simulink model "GFM"  (R2021b)
settings: Solver=ode8  StartTime=0.0  StopTime=5  FixedStep=0.0001  RelTol=1e-3
libraries: spsFirstOrderFilterLib x7, slpidlib x4, spsThreePhaseSeriesRLCBranchLib x4, spsThreePhaseVIMeasurementLib x3, spsabctodq0Lib x3, spsGroundLib x2, rtlab x1, spsCurrentMeasurementLib x1, spsDCVoltageSourceLib x1, spsPower3phInstantaneousLib x1, spsSeriesRLCBranchLib x1, simulink x1
settings Model: Creator=Silov  LastModifiedBy=ti
settings SolverCC: AlgebraicLoopSolver=TrustRegion
settings OptimizationCC: BlockReduction=off  OptimizeBlockIOStorage=off
settings DebuggingCC: SFMachineParentedDataDiag=warning  ArithmeticOperatorsInVariantConditions=warning
settings SFSimCC: CustomCodeUndefinedFunction=UseInterfaceOnly

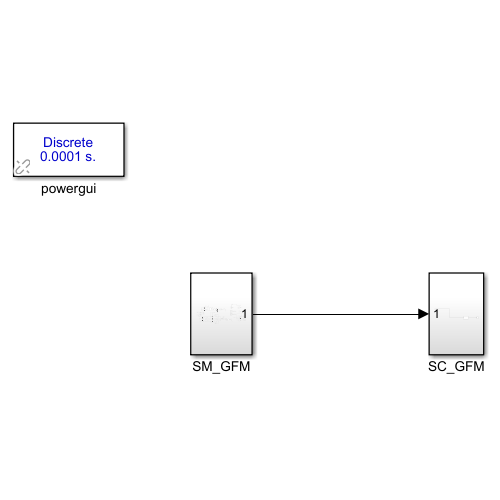
[thumbnail: Simulink's stored preview of the top-level diagram]
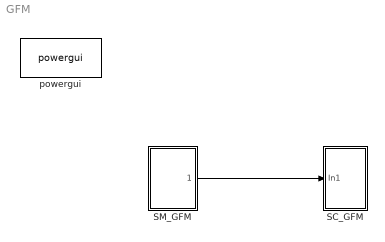
== system GFM ==
  SC_GFM : Subsystem
  SM_GFM : Subsystem
  powergui : spspowerguiLib/powergui  Priority=1  SimulationMode=Discrete  SampleTime=0.0001  frequency=60  Iterations=50  frequencyindice=0  Pbase=100e6  ErrMax=1e-4  UnitsV=kV  UnitsW=MW  buscounter=0  FunctionMessages=off  echomessages=off  EnableUseOfTLC=off  CurrentSourceSwitches=off  DisableSnubberDevices=off  DisableRonSwitches=off  DisableVfSwitches=off  DisplayEquations=off  AutomaticDiscreteSolvers=off  SolverType=Tustin/Backward Euler (TBE)  Interpol=off  ExternalGateDelay=off  methode=off  Ts=100  x0status=blocks  SPID=off  SwTol=0  HookPort=off  NonlinearTolerance=1e-4  nMaxIteration=100  ContinueOnMaxIteration=off  RestoreLinks=warning  ResistiveCurrentMeasurement=off  Frange=[0:2:500]  Ylog=off  Xlog=on  ShowGrid=off  save=off  variable=ZData  structure=grid_current  ZoomFFT=off  StartTime=0.5  cycles=1  DisplayStyle=2  fundamental=50  FreqAxis=off  MaxFrequency=1000  frequencyindicesteady=1  RmsSteady=1  display=off
  wires:
  SM_GFM/1(Outport) -> SC_GFM/1(In1)

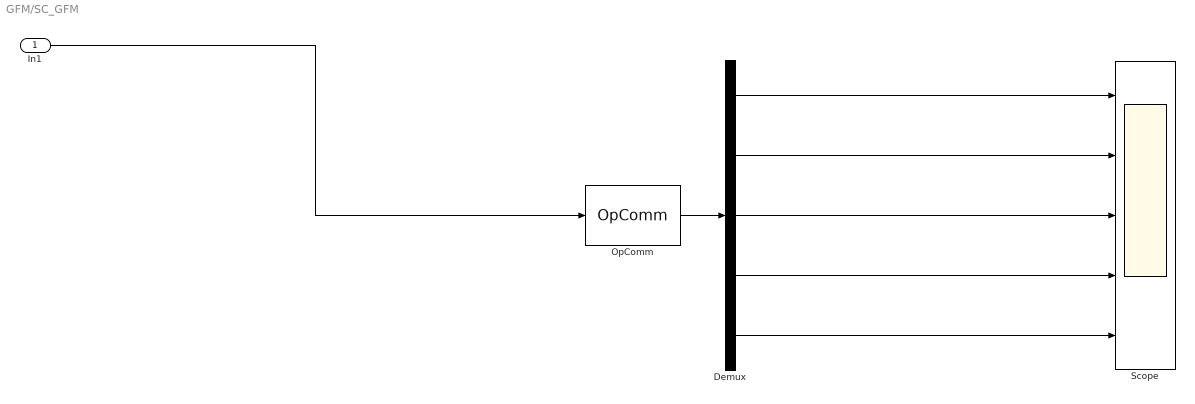
== system GFM/SC_GFM ==
  In1 : Inport
  Demux : Demux  Outputs=5
  OpComm : rtlab/OpComm  nbport=1  groupe_acq=1  subsys_rate=0  st=0  Synchronization=on  Interpolation=on  Threshold=1.0  Missed_Data=off  Sim_Time=off  Samples=off  dynSigOut=off  from_console=0  warning_done=off  writeOpCommFile=off  Offset=off
      settings: SourceProductName=RT-LAB
  Scope : Scope  NumInputPorts=5
  wires:
  OpComm/1 -> Demux/1
  In1/1 -> OpComm/1
  Demux/1 -> Scope/1
  Demux/2 -> Scope/2
  Demux/3 -> Scope/3
  Demux/4 -> Scope/4
  Demux/5 -> Scope/5

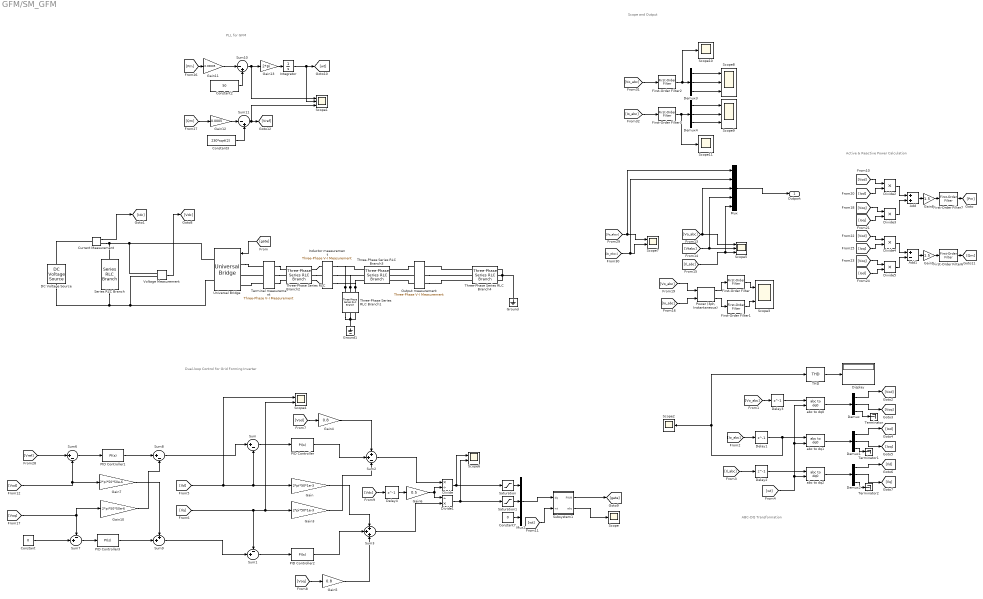
== system GFM/SM_GFM ==
  note: Dual-loop Control for Grid Forming Inverter
  note: ABC-DQ Transformation
  note: Active & Reactive Power Calculation
  note: Scope and Output
  note: PLL for GFM
  Add : Sum
  Add1 : Sum  Inputs=+-
  Constant : Constant  Value=0
  Constant2 : Constant  Value=50
  Constant3 : Constant  Value=230*sqrt(2)
  Constant7 : Constant  Value=0
  Current Measurement : spsCurrentMeasurementLib/Current Measurement  PhasorSimulation=off  OutputType=Complex  PSBequivalent=0
  DC Voltage Source : spsDCVoltageSourceLib/DC Voltage Source  Amplitude=750  Measurements=None
  Delay{1..4} (4 alike) : Delay  DelayLength=1
  Demux{,1..4} (5 alike) : Demux  Outputs=3
  Display : Display
  Divide : Product  Inputs=*/
  Divide1 : Product  Inputs=/*
  Divide{2..5} (4 alike) : Product  Inputs=**
  First-Order Filter{,1..3,6..7} (6 alike) : spsFirstOrderFilterLib/First-Order Filter  FilterType=Lowpass  Tc=0.03183  Ts=0  Initialize=off  Vac_Init=[0, 0, 60]  Vdc_Init=0  PlotResponse=off  FreqRange="[0,  200,  1]"
  Gain : Gain  Gain=2*pi*50*1e-3
  Gain10 : Gain  Gain=2*pi*50*50e-6
  Gain11 : Gain  Gain=0.00005
  Gain12 : Gain  Gain=0.0005
  Gain13 : Gain  Gain=2*pi
  Gain3 : Gain  Gain=2*pi*50*1e-3
  Gain4 : Gain  Gain=0.8
  Gain5 : Gain  Gain=0.8
  Gain6 : Gain  Gain=0.5
  Gain7 : Gain  Gain=2*pi*50*50e-6
  Gain8 : Gain  Gain=1.5
  Gain9 : Gain  Gain=1.5
  Ground : spsGroundLib/Ground  LConnTagsString=a
  Ground1 : spsGroundLib/Ground  LConnTagsString=a
  Inductor measurement : spsThreePhaseVIMeasurementLib/Three-Phase V-I Measurement  VoltageMeasurement=phase-to-ground  SetLabelV=on  LabelV=Vl_abc  Vpu=off  VpuLL=off  CurrentMeasurement=yes  SetLabelI=on  LabelI=Il_abc  Ipu=off  Pbase=100e6  Vbase=500e3  OutputType=Complex  PhasorSimulation=off  PSBequivalent=0
  Integrator : Integrator  WrapState=on  WrappedStateUpperValue=2*pi  WrappedStateLowerValue=0
  Mux : Mux  Inputs=5
  Mux2 : Mux  Inputs=3
  Output measurement : spsThreePhaseVIMeasurementLib/Three-Phase V-I Measurement  VoltageMeasurement=phase-to-ground  SetLabelV=on  LabelV=Vo_abc  Vpu=off  VpuLL=off  CurrentMeasurement=yes  SetLabelI=on  LabelI=Io_abc  Ipu=off  Pbase=100e6  Vbase=500e3  OutputType=Complex  PhasorSimulation=off  PSBequivalent=0
  PID Controller : slpidlib/PID Controller  Controller=PI  Form=Parallel  TimeDomain=Continuous-time  UseExternalTs=off  SampleTime=-1  IntegratorMethod=Forward Euler  FilterMethod=Forward Euler  ControllerParametersSource=internal  P=2*pi  I=pi*1000  D=0  UseFilter=on  N=100  TunerSelectOption=Transfer Function Based (PID Tuner App)  InitialConditionSource=internal  InitialConditionForIntegrator=0  InitialConditionForFilter=0  DifferentiatorICPrevScaledInput=0  ExternalReset=none  TrackingMode=off  Kt=1  LimitOutput=off  SatLimitsSource=internal  UpperSaturationLimit=inf  LowerSaturationLimit=-inf  LinearizeAsGain=on  AntiWindupMode=none  Kb=1  POutMin=[]  POutMax=[]  IOutMin=[]  IOutMax=[]  DOutMin=[]  DOutMax=[]  NOutMin=[]  NOutMax=[]  SumOutMin=[]  SumOutMax=[]  SaturationOutMin=[]  SaturationOutMax=[]  PParamMin=[]  PParamMax=[]  IParamMin=[]  IParamMax=[]  DParamMin=[]  DParamMax=[]  NParamMin=[]  NParamMax=[]  KbParamMin=[]  KbParamMax=[]  KtParamMin=[]  KtParamMax=[]  KbOutMin=[]  KbOutMax=[]  KtOutMin=[]  KtOutMax=[]  IntegratorOutMin=[]  IntegratorOutMax=[]  FilterOutMin=[]  FilterOutMax=[]  SumI1OutMin=[]  SumI1OutMax=[]  SumI2OutMin=[]  SumI2OutMax=[]  SumI3OutMin=[]  SumI3OutMax=[]  SumI4OutMin=[]  SumI4OutMax=[]  SumDOutMin=[]  SumDOutMax=[]  DifferentiatorOutMin=[]  DifferentiatorOutMax=[]  FilterDiffOutCoefMin=[]  FilterDiffOutCoefMax=[]  ReciprocalOutMin=[]  ReciprocalOutMax=[]  SumDenOutMin=[]  SumDenOutMax=[]  SumNumOutMin=[]  SumNumOutMax=[]  DivideOutMin=[]  DivideOutMax=[]  UdiffTsProdOutMin=[]  UdiffTsProdOutMax=[]  NTsProdOutMin=[]  NTsProdOutMax=[]  UintegralTsProdOutMin=[]  UintegralTsProdOutMax=[]  UngainTsProdOutMin=[]  UngainTsProdOutMax=[]  FilterDenConstantOutDataTypeStr=Inherit: Inherit via back propagation  FilterDenConstantOutMin=[]  FilterDenConstantOutMax=[]  PCopyOutDataTypeStr=Inherit: Inherit via back propagation  PCopyOutMin=[]  PCopyOutMax=[]  NCopyOutDataTypeStr=Inherit: Inherit via back propagation  NCopyOutMin=[]  NCopyOutMax=[]  IntegratorContinuousStateAttributes=''  IntegratorStateMustResolveToSignalObject=off  IntegratorRTWStateStorageClass=Auto  FilterContinuousStateAttributes=''  FilterStateMustResolveToSignalObject=off  FilterRTWStateStorageClass=Auto  ParallelPVariant=InternalParameters  IdealPVariant=Disabled  IVariant=InternalParameters  DVariant=Disabled  IntegratorVariant=Continuous  SatVariant=Disabled  AWVariant=Passthrough  PCopyVariant=Disabled  TRVariant=Disabled  FdbkBlocksVariant=Forward  IdealPFdbkVariant=Disabled  SatFdbkVariant=Disabled  DerivativeFilterVariant=Disabled  NVariant=Disabled  NCopyVariant=Disabled_SignalSpec  FilterICVariant=Disabled  IntegratorICVariant=InternalICs  ExternalResetVariant=Disabled  TRSumVariant=Passthrough  SumFdbkVariant=Disabled  SumVariant=Sum_PI  TsampFilterVariant=InternalTs  TsampNgainVariant=Passthrough  TsampIntegralVariant=Passthrough  ExternalSaturationOutDataTypeStr=Inherit: Same as second input
  PID Controller1 : slpidlib/PID Controller  Controller=PI  Form=Parallel  TimeDomain=Continuous-time  UseExternalTs=off  SampleTime=-1  IntegratorMethod=Forward Euler  FilterMethod=Forward Euler  ControllerParametersSource=internal  P=pi/100  I=20*pi  D=0  UseFilter=on  N=100  TunerSelectOption=Transfer Function Based (PID Tuner App)  InitialConditionSource=internal  InitialConditionForIntegrator=0  InitialConditionForFilter=0  DifferentiatorICPrevScaledInput=0  ExternalReset=none  TrackingMode=off  Kt=1  LimitOutput=off  SatLimitsSource=internal  UpperSaturationLimit=inf  LowerSaturationLimit=-inf  LinearizeAsGain=on  AntiWindupMode=none  Kb=1  POutMin=[]  POutMax=[]  IOutMin=[]  IOutMax=[]  DOutMin=[]  DOutMax=[]  NOutMin=[]  NOutMax=[]  SumOutMin=[]  SumOutMax=[]  SaturationOutMin=[]  SaturationOutMax=[]  PParamMin=[]  PParamMax=[]  IParamMin=[]  IParamMax=[]  DParamMin=[]  DParamMax=[]  NParamMin=[]  NParamMax=[]  KbParamMin=[]  KbParamMax=[]  KtParamMin=[]  KtParamMax=[]  KbOutMin=[]  KbOutMax=[]  KtOutMin=[]  KtOutMax=[]  IntegratorOutMin=[]  IntegratorOutMax=[]  FilterOutMin=[]  FilterOutMax=[]  SumI1OutMin=[]  SumI1OutMax=[]  SumI2OutMin=[]  SumI2OutMax=[]  SumI3OutMin=[]  SumI3OutMax=[]  SumI4OutMin=[]  SumI4OutMax=[]  SumDOutMin=[]  SumDOutMax=[]  DifferentiatorOutMin=[]  DifferentiatorOutMax=[]  FilterDiffOutCoefMin=[]  FilterDiffOutCoefMax=[]  ReciprocalOutMin=[]  ReciprocalOutMax=[]  SumDenOutMin=[]  SumDenOutMax=[]  SumNumOutMin=[]  SumNumOutMax=[]  DivideOutMin=[]  DivideOutMax=[]  UdiffTsProdOutMin=[]  UdiffTsProdOutMax=[]  NTsProdOutMin=[]  NTsProdOutMax=[]  UintegralTsProdOutMin=[]  UintegralTsProdOutMax=[]  UngainTsProdOutMin=[]  UngainTsProdOutMax=[]  FilterDenConstantOutDataTypeStr=Inherit: Inherit via back propagation  FilterDenConstantOutMin=[]  FilterDenConstantOutMax=[]  PCopyOutDataTypeStr=Inherit: Inherit via back propagation  PCopyOutMin=[]  PCopyOutMax=[]  NCopyOutDataTypeStr=Inherit: Inherit via back propagation  NCopyOutMin=[]  NCopyOutMax=[]  IntegratorContinuousStateAttributes=''  IntegratorStateMustResolveToSignalObject=off  IntegratorRTWStateStorageClass=Auto  FilterContinuousStateAttributes=''  FilterStateMustResolveToSignalObject=off  FilterRTWStateStorageClass=Auto  ParallelPVariant=InternalParameters  IdealPVariant=Disabled  IVariant=InternalParameters  DVariant=Disabled  IntegratorVariant=Continuous  SatVariant=Disabled  AWVariant=Passthrough  PCopyVariant=Disabled  TRVariant=Disabled  FdbkBlocksVariant=Forward  IdealPFdbkVariant=Disabled  SatFdbkVariant=Disabled  DerivativeFilterVariant=Disabled  NVariant=Disabled  NCopyVariant=Disabled_SignalSpec  FilterICVariant=Disabled  IntegratorICVariant=InternalICs  ExternalResetVariant=Disabled  TRSumVariant=Passthrough  SumFdbkVariant=Disabled  SumVariant=Sum_PI  TsampFilterVariant=InternalTs  TsampNgainVariant=Passthrough  TsampIntegralVariant=Passthrough  ExternalSaturationOutDataTypeStr=Inherit: Same as second input
  PID Controller2 : slpidlib/PID Controller  Controller=PI  Form=Parallel  TimeDomain=Continuous-time  UseExternalTs=off  SampleTime=-1  IntegratorMethod=Forward Euler  FilterMethod=Forward Euler  ControllerParametersSource=internal  P=2*pi  I=pi*1000  D=0  UseFilter=on  N=100  TunerSelectOption=Transfer Function Based (PID Tuner App)  InitialConditionSource=internal  InitialConditionForIntegrator=0  InitialConditionForFilter=0  DifferentiatorICPrevScaledInput=0  ExternalReset=none  TrackingMode=off  Kt=1  LimitOutput=off  SatLimitsSource=internal  UpperSaturationLimit=inf  LowerSaturationLimit=-inf  LinearizeAsGain=on  AntiWindupMode=none  Kb=1  POutMin=[]  POutMax=[]  IOutMin=[]  IOutMax=[]  DOutMin=[]  DOutMax=[]  NOutMin=[]  NOutMax=[]  SumOutMin=[]  SumOutMax=[]  SaturationOutMin=[]  SaturationOutMax=[]  PParamMin=[]  PParamMax=[]  IParamMin=[]  IParamMax=[]  DParamMin=[]  DParamMax=[]  NParamMin=[]  NParamMax=[]  KbParamMin=[]  KbParamMax=[]  KtParamMin=[]  KtParamMax=[]  KbOutMin=[]  KbOutMax=[]  KtOutMin=[]  KtOutMax=[]  IntegratorOutMin=[]  IntegratorOutMax=[]  FilterOutMin=[]  FilterOutMax=[]  SumI1OutMin=[]  SumI1OutMax=[]  SumI2OutMin=[]  SumI2OutMax=[]  SumI3OutMin=[]  SumI3OutMax=[]  SumI4OutMin=[]  SumI4OutMax=[]  SumDOutMin=[]  SumDOutMax=[]  DifferentiatorOutMin=[]  DifferentiatorOutMax=[]  FilterDiffOutCoefMin=[]  FilterDiffOutCoefMax=[]  ReciprocalOutMin=[]  ReciprocalOutMax=[]  SumDenOutMin=[]  SumDenOutMax=[]  SumNumOutMin=[]  SumNumOutMax=[]  DivideOutMin=[]  DivideOutMax=[]  UdiffTsProdOutMin=[]  UdiffTsProdOutMax=[]  NTsProdOutMin=[]  NTsProdOutMax=[]  UintegralTsProdOutMin=[]  UintegralTsProdOutMax=[]  UngainTsProdOutMin=[]  UngainTsProdOutMax=[]  FilterDenConstantOutDataTypeStr=Inherit: Inherit via back propagation  FilterDenConstantOutMin=[]  FilterDenConstantOutMax=[]  PCopyOutDataTypeStr=Inherit: Inherit via back propagation  PCopyOutMin=[]  PCopyOutMax=[]  NCopyOutDataTypeStr=Inherit: Inherit via back propagation  NCopyOutMin=[]  NCopyOutMax=[]  IntegratorContinuousStateAttributes=''  IntegratorStateMustResolveToSignalObject=off  IntegratorRTWStateStorageClass=Auto  FilterContinuousStateAttributes=''  FilterStateMustResolveToSignalObject=off  FilterRTWStateStorageClass=Auto  ParallelPVariant=InternalParameters  IdealPVariant=Disabled  IVariant=InternalParameters  DVariant=Disabled  IntegratorVariant=Continuous  SatVariant=Disabled  AWVariant=Passthrough  PCopyVariant=Disabled  TRVariant=Disabled  FdbkBlocksVariant=Forward  IdealPFdbkVariant=Disabled  SatFdbkVariant=Disabled  DerivativeFilterVariant=Disabled  NVariant=Disabled  NCopyVariant=Disabled_SignalSpec  FilterICVariant=Disabled  IntegratorICVariant=InternalICs  ExternalResetVariant=Disabled  TRSumVariant=Passthrough  SumFdbkVariant=Disabled  SumVariant=Sum_PI  TsampFilterVariant=InternalTs  TsampNgainVariant=Passthrough  TsampIntegralVariant=Passthrough  ExternalSaturationOutDataTypeStr=Inherit: Same as second input
  PID Controller3 : slpidlib/PID Controller  Controller=PI  Form=Parallel  TimeDomain=Continuous-time  UseExternalTs=off  SampleTime=-1  IntegratorMethod=Forward Euler  FilterMethod=Forward Euler  ControllerParametersSource=internal  P=pi/100  I=20*pi  D=0  UseFilter=on  N=100  TunerSelectOption=Transfer Function Based (PID Tuner App)  InitialConditionSource=internal  InitialConditionForIntegrator=0  InitialConditionForFilter=0  DifferentiatorICPrevScaledInput=0  ExternalReset=none  TrackingMode=off  Kt=1  LimitOutput=off  SatLimitsSource=internal  UpperSaturationLimit=inf  LowerSaturationLimit=-inf  LinearizeAsGain=on  AntiWindupMode=none  Kb=1  POutMin=[]  POutMax=[]  IOutMin=[]  IOutMax=[]  DOutMin=[]  DOutMax=[]  NOutMin=[]  NOutMax=[]  SumOutMin=[]  SumOutMax=[]  SaturationOutMin=[]  SaturationOutMax=[]  PParamMin=[]  PParamMax=[]  IParamMin=[]  IParamMax=[]  DParamMin=[]  DParamMax=[]  NParamMin=[]  NParamMax=[]  KbParamMin=[]  KbParamMax=[]  KtParamMin=[]  KtParamMax=[]  KbOutMin=[]  KbOutMax=[]  KtOutMin=[]  KtOutMax=[]  IntegratorOutMin=[]  IntegratorOutMax=[]  FilterOutMin=[]  FilterOutMax=[]  SumI1OutMin=[]  SumI1OutMax=[]  SumI2OutMin=[]  SumI2OutMax=[]  SumI3OutMin=[]  SumI3OutMax=[]  SumI4OutMin=[]  SumI4OutMax=[]  SumDOutMin=[]  SumDOutMax=[]  DifferentiatorOutMin=[]  DifferentiatorOutMax=[]  FilterDiffOutCoefMin=[]  FilterDiffOutCoefMax=[]  ReciprocalOutMin=[]  ReciprocalOutMax=[]  SumDenOutMin=[]  SumDenOutMax=[]  SumNumOutMin=[]  SumNumOutMax=[]  DivideOutMin=[]  DivideOutMax=[]  UdiffTsProdOutMin=[]  UdiffTsProdOutMax=[]  NTsProdOutMin=[]  NTsProdOutMax=[]  UintegralTsProdOutMin=[]  UintegralTsProdOutMax=[]  UngainTsProdOutMin=[]  UngainTsProdOutMax=[]  FilterDenConstantOutDataTypeStr=Inherit: Inherit via back propagation  FilterDenConstantOutMin=[]  FilterDenConstantOutMax=[]  PCopyOutDataTypeStr=Inherit: Inherit via back propagation  PCopyOutMin=[]  PCopyOutMax=[]  NCopyOutDataTypeStr=Inherit: Inherit via back propagation  NCopyOutMin=[]  NCopyOutMax=[]  IntegratorContinuousStateAttributes=''  IntegratorStateMustResolveToSignalObject=off  IntegratorRTWStateStorageClass=Auto  FilterContinuousStateAttributes=''  FilterStateMustResolveToSignalObject=off  FilterRTWStateStorageClass=Auto  ParallelPVariant=InternalParameters  IdealPVariant=Disabled  IVariant=InternalParameters  DVariant=Disabled  IntegratorVariant=Continuous  SatVariant=Disabled  AWVariant=Passthrough  PCopyVariant=Disabled  TRVariant=Disabled  FdbkBlocksVariant=Forward  IdealPFdbkVariant=Disabled  SatFdbkVariant=Disabled  DerivativeFilterVariant=Disabled  NVariant=Disabled  NCopyVariant=Disabled_SignalSpec  FilterICVariant=Disabled  IntegratorICVariant=InternalICs  ExternalResetVariant=Disabled  TRSumVariant=Passthrough  SumFdbkVariant=Disabled  SumVariant=Sum_PI  TsampFilterVariant=InternalTs  TsampNgainVariant=Passthrough  TsampIntegralVariant=Passthrough  ExternalSaturationOutDataTypeStr=Inherit: Same as second input
  "Power (3ph, Instantaneous)" : spsPower3phInstantaneousLib/Power (3ph, Instantaneous)
  Saturation : Saturate  UpperLimit=1  LowerLimit=-1
  Saturation1 : Saturate  UpperLimit=1  LowerLimit=-1
  Scope{,2,10..11} (4 alike) : Scope
  Scope{1,5,8..9} (4 alike) : Scope  NumInputPorts=3
  Scope{3..4,6..7} (4 alike) : Scope  NumInputPorts=2
  Series RLC Branch : spsSeriesRLCBranchLib/Series RLC Branch  LConnTagsString=__new0  RConnTagsString=__new0  BranchType=RC  Resistance=0.005  Inductance=1e-3  SetiL0=off  InitialCurrent=0  Capacitance=1000e-6  Setx0=on  InitialVoltage=750  Measurements=None
  Subsystem1 : Subsystem  mask{rep_seq_t=[0 1/4 2/4 3/4 4/4]./10000}
      mask prompts: rep_seq_t "Simulink:masks:TimeValues_MP"
      mask TypeOptions rep_seq_t:
      | Repeating
      | Sequence1/rep_seq_t
      mask DialogControl rep_seq_t Prompt: Time values:
  Sum : Sum  Inputs=|+-
  Sum1 : Sum  Inputs=-+|
  Sum10 : Sum  Inputs=|-+
  Sum11 : Sum  Inputs=|-+
  Sum2 : Sum  Inputs=++-
  Sum3 : Sum  Inputs=+++
  Sum6 : Sum  Inputs=|+-
  Sum7 : Sum  Inputs=-+|
  Sum8 : Sum  Inputs=|+-
  Sum9 : Sum  Inputs=++|
  THD : spsTHDLib/THD  Freq=50  Ts=0
      settings: SourceProductBaseCode=PS
  Terminal measurement : spsThreePhaseVIMeasurementLib/Three-Phase V-I Measurement  VoltageMeasurement=phase-to-ground  SetLabelV=on  LabelV=Vtabc  Vpu=off  VpuLL=off  CurrentMeasurement=yes  SetLabelI=on  LabelI=Itabc  Ipu=off  Pbase=100e6  Vbase=500e3  OutputType=Complex  PhasorSimulation=off  PSBequivalent=0
  Terminator : Terminator
  Terminator1 : Terminator
  Terminator2 : Terminator
  Three-Phase Series RLC Branch1 : spsThreePhaseSeriesRLCBranchLib/Three-Phase Series RLC Branch  LConnTagsString=A|B|C  RConnTagsString=A|B|C  BranchType=C  Resistance=0.05  Inductance=4e-3  Capacitance=50e-6  Measurements=None
  Three-Phase Series RLC Branch2 : spsThreePhaseSeriesRLCBranchLib/Three-Phase Series RLC Branch  LConnTagsString=A|B|C  RConnTagsString=A|B|C  BranchType=RL  Resistance=0.2  Inductance=1e-3  Capacitance=1e-6  Measurements=None
  Three-Phase Series RLC Branch3 : spsThreePhaseSeriesRLCBranchLib/Three-Phase Series RLC Branch  LConnTagsString=A|B|C  RConnTagsString=A|B|C  BranchType=RL  Resistance=0.3  Inductance=300e-6  Capacitance=1e-6  Measurements=None
  Three-Phase Series RLC Branch4 : spsThreePhaseSeriesRLCBranchLib/Three-Phase Series RLC Branch  LConnTagsString=A|B|C  RConnTagsString=A|B|C  BranchType=R  Resistance=20  Inductance=300e-6  Capacitance=1e-6  Measurements=None
  Universal Bridge : spsUniversalBridgeLib/Universal Bridge  Arms=3  SnubberResistance=1e5  SnubberCapacitance=inf  Device=IGBT / Diodes  Ron=1e-3  Lon=0  ForwardVoltages="[  0  0  ]"  ForwardVoltage=0  GTOparameters=[ 10e-6 , 20e-6 ]  IGBTparameters=[ 1e-6 , 2e-6 ]  Measurements=None  Measurements_2=None  converterType=Rectifier
  Voltage Measurement : spsVoltageMeasurementLib/Voltage Measurement  PhasorSimulation=off  OutputType=Complex  PSBequivalent=0
  abc to dq0 : spsabctodq0Lib/abc to dq0  Alignment=90 degrees behind phase A axis
  abc to dq1 : spsabctodq0Lib/abc to dq0  Alignment=90 degrees behind phase A axis
  abc to dq2 : spsabctodq0Lib/abc to dq0  Alignment=90 degrees behind phase A axis
  Outport : Outport  VectorParamsAs1DForOutWhenUnconnected=off
  wires:
  PID Controller1/1 -> Sum8/1
  Demux2/2 -> [Ilq]
  First-Order Filter7/1 -> [Pm]
  Delay3/1 -> abc to dq0/1
  Divide1/1 -> Scope6/2, Saturation1/1
  [Ild] -> Sum/2, Gain/1, Scope4/1
  Integrator/1 -> Scope1/2, [wt]
  abc to dq1/1 -> Demux1/1
  First-Order Filter6/1 -> [Qm]
  [Io_abcx] -> Mux/2, Scope7/2
  [Vo_abc] -> Mux/3, Scope5/1
  [Pm] -> Gain11/1
  Gain6/1 -> Divide1/1, Divide/2
  THD/1 -> Display/1
  Gain/1 -> Sum3/1
  Demux2/3 -> Terminator2/1
  [Vo_abc] -> "Power (3ph, Instantaneous)"/1
  First-Order Filter1/1 -> Scope3/2
  [wt] -> abc to dq0/2, abc to dq1/2, abc to dq2/2
  [gate] -> Universal Bridge/1
  abc to dq2/1 -> Demux2/1
  abc to dq0/1 -> Demux/1
  Gain7/1 -> Sum9/1
  Sum9/1 -> Sum1/2
  Divide/1 -> Saturation/1, Scope6/1
  Sum10/1 -> Scope1/1, Gain13/1
  Current Measurement/1 -> [Idc]
  "Power (3ph, Instantaneous)"/1 -> First-Order Filter/1
  Sum1/1 -> PID Controller2/1
  Demux/2 -> [Voq]
  [Voq] -> Divide5/1
  Constant7/1 -> Mux2/3
  Gain4/1 -> Sum2/1
  [wt] -> Subsystem1/2(wt)
  Sum/1 -> PID Controller/1
  [Vtabc] -> Mux/4, Scope5/2
  [Il_abc] -> Delay2/1
  Delay1/1 -> THD/1, Scope2/1, abc to dq1/1
  Demux/3 -> Terminator/1
  [Vref] -> Sum6/1
  PID Controller2/1 -> Sum3/2
  [Io_abc] -> Delay1/1
  [Io_abc] -> "Power (3ph, Instantaneous)"/2
  [Il_abc] -> Mux/5, Scope5/3
  Gain10/1 -> Sum8/2
  Sum2/1 -> Divide/1
  Demux1/2 -> [Ioq]
  Subsystem1/1(PWM) -> [gate]
  Mux2/1 -> Subsystem1/1(dq)
  PID Controller3/1 -> Sum9/2
  [Vdc] -> Delay4/1
  [Voq] -> Gain5/1
  Demux/1 -> [Vod]
  Divide4/1 -> Add1/1
  [Voq] -> Divide3/1
  [Ioq] -> Divide3/2
  [Vod] -> Sum6/2, Gain7/1
  [Vod] -> Divide2/1
  Demux2/1 -> [Ild]
  Sum7/1 -> PID Controller3/1
  Sum6/1 -> PID Controller1/1
  Sum11/1 -> Scope1/3, [Vref]
  "Power (3ph, Instantaneous)"/2 -> First-Order Filter1/1
  Voltage Measurement/1 -> [Vdc]
  [Vod] -> Divide4/1
  Gain8/1 -> First-Order Filter7/1
  Delay4/1 -> Gain6/1
  Add1/1 -> Gain9/1
  Divide5/1 -> Add1/2
  Divide2/1 -> Add/1
  Gain9/1 -> First-Order Filter6/1
  Saturation/1 -> Mux2/1
  [Ioq] -> Divide4/2
  [Qm] -> Gain12/1
  Add/1 -> Gain8/1
  Divide3/1 -> Add/2
  Gain5/1 -> Sum3/3
  Sum3/1 -> Divide1/2
  Gain3/1 -> Sum2/3
  Gain13/1 -> Integrator/1
  [Iod] -> Divide5/2
  Gain11/1 -> Sum10/1
  [Vod] -> Gain4/1
  Constant/1 -> Sum7/2
  Delay2/1 -> abc to dq2/1
  Gain12/1 -> Sum11/1
  Demux1/3 -> Terminator1/1
  Constant2/1 -> Sum10/2
  [Ilq] -> Scope4/2, Gain3/1, Sum1/1
  [Iod] -> Divide2/2
  Demux1/1 -> [Iod]
  [Vo_abc] -> Delay3/1
  First-Order Filter/1 -> Scope3/1
  Sum8/1 -> Sum/1
  Saturation1/1 -> Mux2/2
  PID Controller/1 -> Sum2/2
  Constant3/1 -> Sum11/2
  [Voq] -> Gain10/1, Sum7/1
  Mux/1 -> Outport/1
  [Vo_abcx] -> Mux/1, Scope7/1
  Subsystem1/2(abc) -> Scope/1
  Demux3/1 -> Scope8/1
  Demux3/2 -> Scope8/2
  Demux3/3 -> Scope8/3
  Demux4/1 -> Scope9/1
  Demux4/2 -> Scope9/2
  Demux4/3 -> Scope9/3
  [Vo_abc] -> First-Order Filter2/1
  First-Order Filter2/1 -> Scope10/1, Demux3/1
  [Io_abc] -> First-Order Filter3/1
  First-Order Filter3/1 -> Scope11/1, Demux4/1
  connections:
  Terminal measurement/RConn3 -- Three-Phase Series RLC Branch2/LConn3
  Output measurement/LConn2 -- Three-Phase Series RLC Branch3/RConn2
  DC Voltage Source/LConn1 -- Voltage Measurement/LConn2 -- Universal Bridge/RConn2 -- Series RLC Branch/RConn1
  Three-Phase Series RLC Branch2/RConn1 -- Inductor measurement/LConn1
  Current Measurement/RConn1 -- Voltage Measurement/LConn1 -- Universal Bridge/RConn1 -- Series RLC Branch/LConn1
  Terminal measurement/RConn1 -- Three-Phase Series RLC Branch2/LConn1
  Three-Phase Series RLC Branch1/LConn1 -- Three-Phase Series RLC Branch3/LConn1 -- Inductor measurement/RConn1
  Three-Phase Series RLC Branch1/LConn2 -- Three-Phase Series RLC Branch3/LConn2 -- Inductor measurement/RConn2
  Output measurement/LConn1 -- Three-Phase Series RLC Branch3/RConn1
  Output measurement/LConn3 -- Three-Phase Series RLC Branch3/RConn3
  Three-Phase Series RLC Branch2/RConn3 -- Inductor measurement/LConn3
  Three-Phase Series RLC Branch1/RConn2 -- Ground1/LConn1 -- Three-Phase Series RLC Branch1/RConn3 -- Three-Phase Series RLC Branch1/RConn1
  Terminal measurement/RConn2 -- Three-Phase Series RLC Branch2/LConn2
  Three-Phase Series RLC Branch1/LConn3 -- Three-Phase Series RLC Branch3/LConn3 -- Inductor measurement/RConn3
  Terminal measurement/LConn3 -- Universal Bridge/LConn3
  Output measurement/RConn3 -- Three-Phase Series RLC Branch4/LConn3
  Current Measurement/LConn1 -- DC Voltage Source/RConn1
  Three-Phase Series RLC Branch4/RConn2 -- Ground/LConn1 -- Three-Phase Series RLC Branch4/RConn1 -- Three-Phase Series RLC Branch4/RConn3
  Output measurement/RConn2 -- Three-Phase Series RLC Branch4/LConn2
  Universal Bridge/LConn1 -- Terminal measurement/LConn1
  Three-Phase Series RLC Branch4/LConn1 -- Output measurement/RConn1
  Three-Phase Series RLC Branch2/RConn2 -- Inductor measurement/LConn2
  Terminal measurement/LConn2 -- Universal Bridge/LConn2

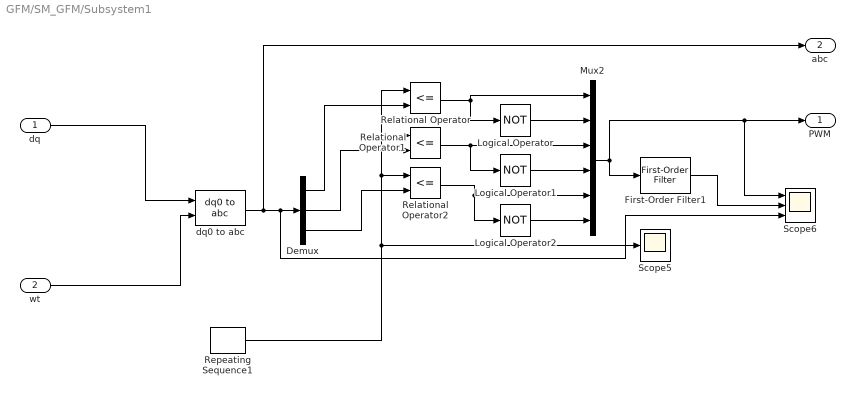
== system GFM/SM_GFM/Subsystem1 ==
  dq : Inport
  wt : Inport  Port=2
  Demux : Demux  Outputs=3
  First-Order Filter1 : spsFirstOrderFilterLib/First-Order Filter  FilterType=Lowpass  Tc=10e-5  Ts=0  Initialize=off  Vac_Init=[0, 0, 60]  Vdc_Init=0  PlotResponse=off  FreqRange="[0,  200,  1]"
  Logical Operator : Logic  Operator=NOT  AllPortsSameDT=off  OutDataTypeStr=boolean
  Logical Operator1 : Logic  Operator=NOT  AllPortsSameDT=off  OutDataTypeStr=boolean
  Logical Operator2 : Logic  Operator=NOT  AllPortsSameDT=off  OutDataTypeStr=boolean
  Mux2 : Mux  Inputs=6
  Relational Operator : RelationalOperator  Operator=<=  OutDataTypeStr=boolean  RndMeth=Simplest
  Relational Operator1 : RelationalOperator  Operator=<=  OutDataTypeStr=boolean  RndMeth=Simplest
  Relational Operator2 : RelationalOperator  Operator=<=  OutDataTypeStr=boolean  RndMeth=Simplest
  Repeating Sequence1 : simulink/Sources/Repeating Sequence  rep_seq_t=rep_seq_t  rep_seq_y=[0 1 0 -1 0]
  Scope5 : Scope
  Scope6 : Scope  NumInputPorts=3
  dq0 to abc : spsdq0toabcLib/dq0 to abc  Alignment=90 degrees behind phase A axis
  PWM : Outport  VectorParamsAs1DForOutWhenUnconnected=off
  abc : Outport  Port=2  VectorParamsAs1DForOutWhenUnconnected=off
  wires:
  wt/1 -> dq0 to abc/2
  Demux/2 -> Relational Operator1/2
  Logical Operator1/1 -> Mux2/4
  dq/1 -> dq0 to abc/1
  Relational Operator2/1 -> Mux2/5, Logical Operator2/1
  Relational Operator/1 -> Mux2/1, Logical Operator/1
  dq0 to abc/1 -> abc/1, Scope6/3, Demux/1
  Demux/1 -> Relational Operator/2
  Logical Operator2/1 -> Mux2/6
  Logical Operator/1 -> Mux2/2
  Mux2/1 -> First-Order Filter1/1, Scope6/1, PWM/1
  Repeating Sequence1/1 -> Relational Operator/1, Relational Operator1/1, Relational Operator2/1, Scope5/1
  Relational Operator1/1 -> Mux2/3, Logical Operator1/1
  Demux/3 -> Relational Operator2/2
  First-Order Filter1/1 -> Scope6/2
